simulink model "sim_step"  (R2018b)
settings: Solver=ode4  StartTime=0.0  StopTime=5  FixedStep=0.001  RelTol=1e-3
settings Model: Creator=kawata  LastModifiedBy=kawata

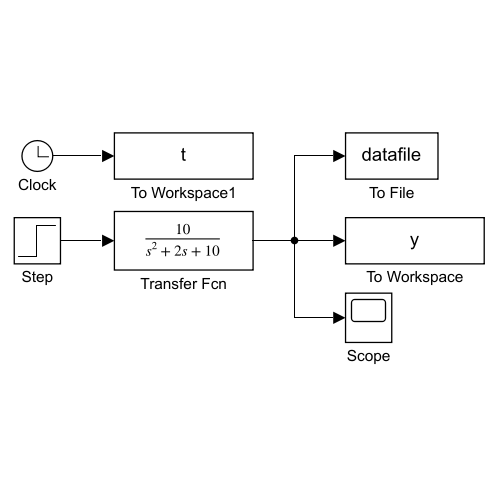
[thumbnail: Simulink's stored preview of the top-level diagram]
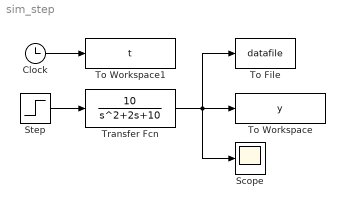
== system sim_step ==
  Clock : Clock
  Scope : Scope
  Step : Step  Time=0  SampleTime=0
  To File : ToFile  Filename=datafile  MatrixName=output  SaveFormat=Timeseries
  To Workspace : ToWorkspace  VariableName=y  SampleTime=-1
  To Workspace1 : ToWorkspace  VariableName=t  SampleTime=-1
  Transfer Fcn : TransferFcn  Numerator=[10]  Denominator=[1 2 10]
  wires:
  Clock/1 -> To Workspace1/1
  Transfer Fcn/1 -> To File/1, Scope/1, To Workspace/1
  Step/1 -> Transfer Fcn/1
